simulink model "fsk"  (R2018b)
settings: Solver=VariableStepAuto  StartTime=0.0  StopTime=10.0  RelTol=1e-3
libraries: dsparch4 x4, commrandsrc3 x1
settings Model: Creator=86138  LastModifiedBy=86138

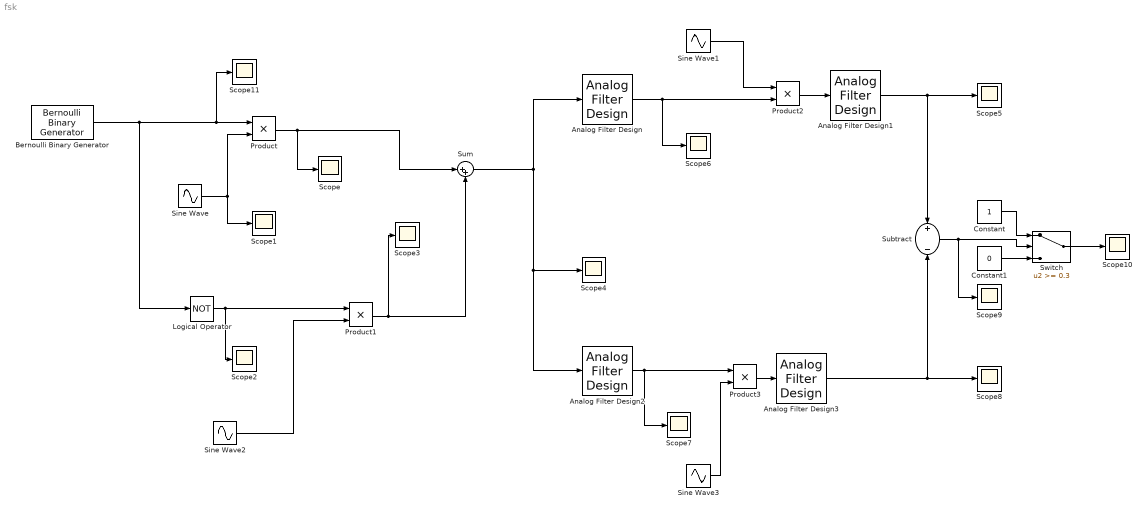
== system fsk ==
  Analog Filter Design : dsparch4/Analog Filter Design  method=Butterworth  filttype=Bandpass  N=8  Wlo=60*pi  Whi=100*pi  Rp=2  Rs=40
  Analog Filter Design1 : dsparch4/Analog Filter Design  method=Butterworth  filttype=Lowpass  N=8  Wlo=10*pi  Whi=80  Rp=2  Rs=40
  Analog Filter Design2 : dsparch4/Analog Filter Design  method=Butterworth  filttype=Bandpass  N=8  Wlo=10*pi  Whi=30*pi  Rp=2  Rs=40
  Analog Filter Design3 : dsparch4/Analog Filter Design  method=Butterworth  filttype=Lowpass  N=8  Wlo=20*pi  Whi=80  Rp=2  Rs=40
  Bernoulli Binary Generator : commrandsrc3/Bernoulli Binary Generator  ProbabilityOfZero=0.5  SeedSource=Auto  Seed=0  SampleTime=1  SamplesPerFrame=1  OutputDataType=double  SimulateUsing=Interpreted execution
  Constant : Constant
  Constant1 : Constant  Value=0
  Logical Operator : Logic  Operator=NOT  AllPortsSameDT=off  OutDataTypeStr=boolean
  Product{,1..3} (4 alike) : Product
  Scope{,1..11} (12 alike) : Scope
  Sine Wave : Sin  Frequency=80*pi  SampleTime=1/500
  Sine Wave1 : Sin  Frequency=80*pi  SampleTime=1/500
  Sine Wave2 : Sin  Frequency=20*pi  SampleTime=1/500
  Sine Wave3 : Sin  Frequency=80*pi  SampleTime=1/500
  Subtract : Sum  Inputs=+-
  Sum : Sum  Inputs=|++
  Switch : Switch  Threshold=0.3
  wires:
  Bernoulli Binary Generator/1 -> Logical Operator/1, Scope11/1, Product/1
  Sine Wave/1 -> Scope1/1, Product/2
  Product/1 -> Sum/1, Scope/1
  Logical Operator/1 -> Scope2/1, Product1/1
  Sine Wave2/1 -> Product1/2
  Product1/1 -> Scope3/1, Sum/2
  Sum/1 -> Analog Filter Design/1, Analog Filter Design2/1, Scope4/1
  Analog Filter Design/1 -> Scope6/1, Product2/2
  Sine Wave1/1 -> Product2/1
  Product2/1 -> Analog Filter Design1/1
  Analog Filter Design1/1 -> Subtract/1, Scope5/1
  Analog Filter Design2/1 -> Scope7/1, Product3/1
  Sine Wave3/1 -> Product3/2
  Product3/1 -> Analog Filter Design3/1
  Analog Filter Design3/1 -> Scope8/1, Subtract/2
  Subtract/1 -> Switch/2, Scope9/1
  Constant1/1 -> Switch/3
  Constant/1 -> Switch/1
  Switch/1 -> Scope10/1
